simulink model "gyro_precession_adjustment"  (R2018b)
settings: Solver=VariableStepAuto  StartTime=0.0  StopTime=10.0  RelTol=1e-3
undefined symbols (not defined in the file): fswParams
libraries: CrossProdMatrix_lib x1
settings Model: Creator=Nick's PC  LastModifiedBy=Nick's PC

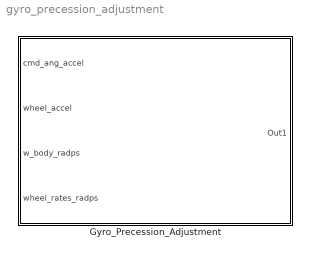
== system gyro_precession_adjustment ==
  Gyro_Precession_Adjustment : Subsystem

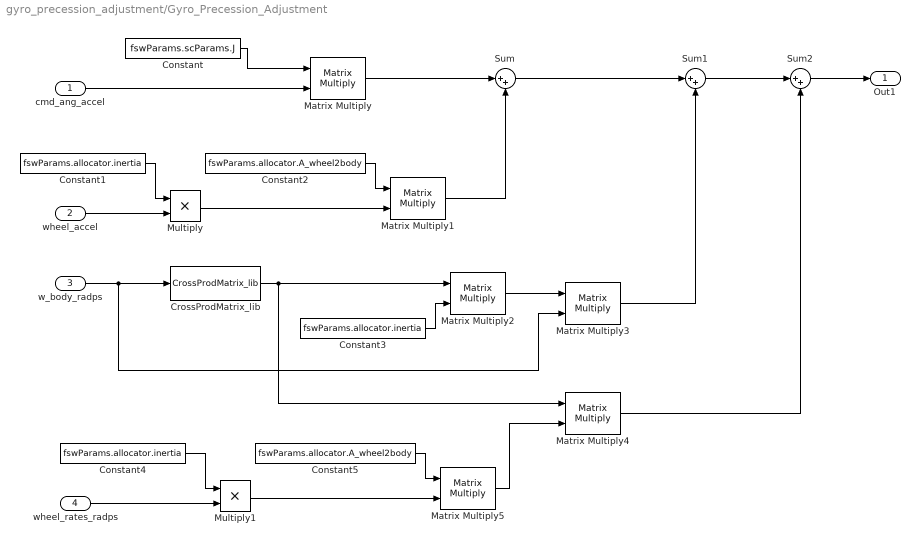
== system gyro_precession_adjustment/Gyro_Precession_Adjustment ==
  cmd_ang_accel : Inport
  wheel_accel : Inport  Port=2
  w_body_radps : Inport  Port=3
  wheel_rates_radps : Inport  Port=4
  Constant : Constant  Value=fswParams.scParams.J
  Constant1 : Constant  Value=fswParams.allocator.inertia
  Constant2 : Constant  Value=fswParams.allocator.A_wheel2body
  Constant3 : Constant  Value=fswParams.allocator.inertia
  Constant4 : Constant  Value=fswParams.allocator.inertia
  Constant5 : Constant  Value=fswParams.allocator.A_wheel2body
  CrossProdMatrix_lib : CrossProdMatrix_lib/CrossProdMatrix_lib  SystemSampleTime=-1
  Matrix Multiply{,1..5} (6 alike) : Product  Multiplication=Matrix(*)
  Multiply : Product
  Multiply1 : Product
  Sum : Sum  Inputs=|++
  Sum1 : Sum  Inputs=|++
  Sum2 : Sum  Inputs=|++
  Out1 : Outport
  wires:
  cmd_ang_accel/1 -> Matrix Multiply/2
  Constant/1 -> Matrix Multiply/1
  Matrix Multiply/1 -> Sum/1
  wheel_accel/1 -> Multiply/2
  Constant1/1 -> Multiply/1
  Multiply/1 -> Matrix Multiply1/2
  Constant2/1 -> Matrix Multiply1/1
  Matrix Multiply1/1 -> Sum/2
  Sum/1 -> Sum1/1
  w_body_radps/1 -> Matrix Multiply3/2, CrossProdMatrix_lib/1
  CrossProdMatrix_lib/1 -> Matrix Multiply4/1, Matrix Multiply2/1
  Constant3/1 -> Matrix Multiply2/2
  Matrix Multiply2/1 -> Matrix Multiply3/1
  Matrix Multiply3/1 -> Sum1/2
  wheel_rates_radps/1 -> Multiply1/2
  Constant5/1 -> Matrix Multiply5/1
  Constant4/1 -> Multiply1/1
  Multiply1/1 -> Matrix Multiply5/2
  Matrix Multiply5/1 -> Matrix Multiply4/2
  Matrix Multiply4/1 -> Sum2/2
  Sum1/1 -> Sum2/1
  Sum2/1 -> Out1/1
